simulink model "mpsk_receiver_simulation"  (Simulink 7.3)
settings: Solver=ode45  StartTime=0.0  StopTime=10.0  RelTol=1e-3
undefined symbols (not defined in the file or in its folder): get
libraries: commsink2 x2, commdigbbndpm3 x1, commphrec2 x1, commtimrec2 x1, commrflib2 x1, dspsrcs4 x1, dspsnks4 x1
settings Model: Creator=joneskoo  LastModifiedBy=joneskoo

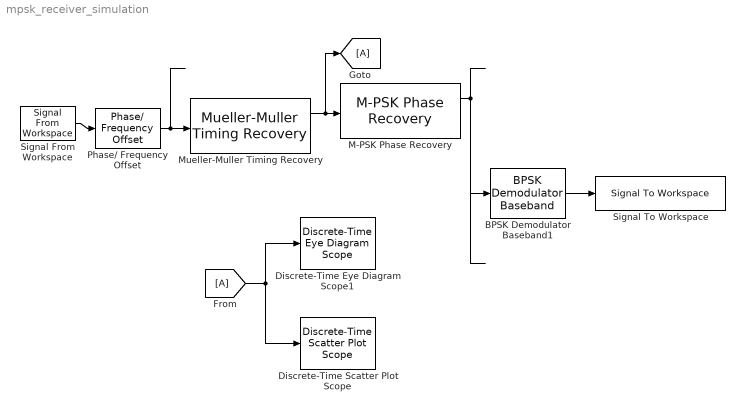
== system mpsk_receiver_simulation ==
  BPSK Demodulator Baseband1 : commdigbbndpm3/BPSK Demodulator Baseband  DialogController=commDDGCreate  DialogControllerArgs=DataTag0  Ph=0  DecType=Hard decision  VarSource=Dialog  Variance=1  outDtype=Inherit via internal rule  derotateFactorWordLen=16
  Discrete-Time Eye Diagram Scope1 : commsink2/Discrete-Time Eye Diagram Scope  Tag=EyeDiagram  SystemSampleTime=-1  sampPerSymb=2  offsetEye=0  symbPerTrace=1  numTraces=100  numNewFrames=50  LineStyles=-  LineColors=b  dupPoints=on  fading=on  render=on  AxisGrid=on  yMin=-3.15  yMax=3.15  inphaseLabel=In-phase Amplitude  quadratureLabel=Quadrature Amplitude  openScopeAtSimStart=on  dispDiagram=In-phase and Quadrature  FrameNumber=off  FigPos=get(0,'defaultfigureposition');  figTitle=Eye Diagram  block_type_=eye  numLinesMax=8
  Discrete-Time Scatter Plot Scope : commsink2/Discrete-Time Scatter Plot Scope  Tag=ScatterPlot  SystemSampleTime=-1  sampPerSymb=1  offsetEye=0  numTraces=40  numNewFrames=20  LineMarkers=.  LineColors=b  fading=on  render=on  AxisGrid=on  xMin=-3.3  xMax=3.315  yMin=-3.3  yMax=3.315  inphaseLabel=In-phase Amplitude  quadratureLabel=Quadrature Amplitude  openScopeAtSimStart=on  FrameNumber=off  FigPos=get(0,'defaultfigureposition');  figTitle=Scatter Plot  numLinesMax=8  block_type_=scatter
  M-PSK Phase Recovery : commphrec2/M-PSK Phase Recovery  SystemSampleTime=-1  M=2  intPeriod=50
  Mueller-Muller Timing Recovery : commtimrec2/Mueller-Muller Timing Recovery  sampPerSymbol=2  propGain=0.05  resetMode=None
  Phase/ Frequency Offset : commrflib2/Phase// Frequency Offset  phaseOffset=27  freqPort=off  freqOffset=0
  Signal From Workspace : dspsrcs4/Signal From Workspace  SystemSampleTime=-1  X=psk_baseband  Ts=1/500000  nsamps=1  OutputAfterFinalValue=Cyclic repetition  ignoreOrWarnInputAndFrameLengths=off
  Signal To Workspace : dspsnks4/Signal To Workspace  SystemSampleTime=-1  VariableName=psk_demod_data  FrameMode=Concatenate frames (2-D array)
      settings: MaxDataPoints=2000  FixptAsFi=off
  wires:
  Signal From Workspace/1 -> Phase/ Frequency Offset/1
  BPSK Demodulator Baseband1/1 -> Signal To Workspace/1
  Phase/ Frequency Offset/1 -> Mueller-Muller Timing Recovery/1
  Mueller-Muller Timing Recovery/1 -> M-PSK Phase Recovery/1, [A]
  M-PSK Phase Recovery/1 -> BPSK Demodulator Baseband1/1
  [A] -> Discrete-Time Eye Diagram Scope1/1, Discrete-Time Scatter Plot Scope/1
